simulink model "Sample2"  (R2020a)
settings: Solver=FixedStepAuto  StartTime=0.0  StopTime=Inf  RelTol=1e-3
settings Model: Creator=eisuk  LastModifiedBy=eisuk
settings SolverCC: PositivePriorityOrder=on
settings DataIOCC: ReturnWorkspaceOutputs=off
settings OptimizationCC: EnhancedBackFolding=on  PassReuseOutputArgsAs=Individual arguments  ZeroExternalMemoryAtStartup=off  ZeroInternalMemoryAtStartup=off  MaxStackSize=64  OptimizeBlockOrder=speed  DifferentSizesBufferReuse=on  OptimizationCustomize=off  EfficientTunableParamExpr=on
settings DebuggingCC: ParameterTunabilityLossMsg=error
settings HardwareCC: ProdBitPerPointer=32  ProdBitPerSizeT=32  ProdBitPerPtrDiffT=32  ProdLargestAtomicInteger=Long  ProdLargestAtomicFloat=Double  ProdWordSize=32  ProdLongLongMode=on  ProdHWDeviceType=ARM Compatible->ARM Cortex
settings RTWCC: SystemTargetFile=ert.tlc  HardwareBoard=Raspberry Pi  TemplateMakefile=ert_default_tmf  Toolchain=GNU GCC Raspberry Pi  BuildConfiguration=Faster Runs
settings CodeAppCC: ForceParamTrailComments=on  IgnoreCustomStorageClasses=off  OperatorAnnotations=on  SimulinkDataObjDesc=on  SFDataObjDesc=on  InsertBlockDesc=on
settings ERTTargetCC: SupportVariableSizeSignals=on

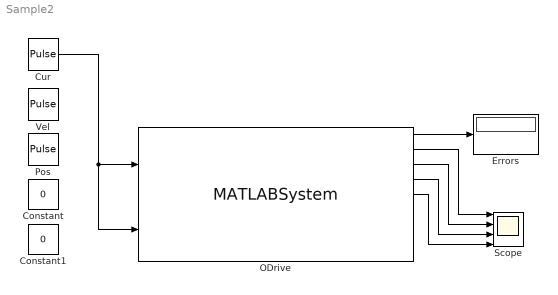
== system Sample2 ==
  Constant : Constant  Value=0
  Constant1 : Constant  Value=0
  Cur : DiscretePulseGenerator  Period=100  PulseWidth=50  PhaseDelay=1  SampleTime=0.1
  Errors : Display
      settings: Format=hex (Stored Integer)
  ODrive : MATLABSystem  System=ODriveRasPi  SampleTime=0.0025  isPort=off  portName=/dev/ttyS0  serial=2059387F304E  isAxis0=on  ctrlMode0=Current  isInCpr0=off  isVelRamp0=off  watchdog0=0  isExternal0=off  posGain0=1  velGain0=0.0001  velIGain0=0.001  velLimit0=200000  velLimitTol0=1.2  velRampRate0=10000.0  isAxis1=on  ctrlMode1=Current  isInCpr1=off  isVelRamp1=off  watchdog1=0  isExternal1=off  posGain1=1  velGain1=0.0001  velIGain1=0.001  velLimit1=200000.0  velLimitTol1=1.2  velRampRate1=10000.0
      mask Type: ODriveRasPi
      mask Display:
      | disp(['ODrive' char(10) '' char(10) 'Serial: 2059387F304E' char(10) '' char(10) 'M0: Current control' char(10) 'M1: Current control']);
      | port_label('input',1,'M0 current ref');
      | port_label('input',2,'M1 current ref');
      | port_label('output',1,'Axis error');
      | port_label('output',2,'M0 position act');
      | port_label('output',3,'M0 velocity act');
      | port_label('output',4,'M0 current act');
      | port_label('output',5,'M0 vel integral act');
      | port_label('output',6,'M1 position act');
      | port_label('output',7,'M1 velocity act');
      | port_label('output',8,'M1 current act');
      | port_label('output',9,'M1 vel integral act');
  Pos : DiscretePulseGenerator  Amplitude=500000  Period=100  PulseWidth=50  PhaseDelay=1  SampleTime=0.1
  Scope : Scope  NumInputPorts=4
  Vel : DiscretePulseGenerator  Amplitude=100000  Period=100  PulseWidth=50  PhaseDelay=1  SampleTime=0.1
  wires:
  ODrive/1 -> Errors/1
  ODrive/2 -> Scope/1
  ODrive/3 -> Scope/2
  ODrive/5 -> Scope/4
  ODrive/4 -> Scope/3
  Cur/1 -> ODrive/2, ODrive/1
